simulink model "pv_test"  (R2016a)
settings: Solver=VariableStepAuto  StartTime=0.0  StopTime=0.02  RelTol=1e-3
libraries: powerlib x99, powerlib_meascontrol x30, re_lib x3, simulink x1
settings Model: Creator=Francis Chen  LastModifiedBy=Francis Chen

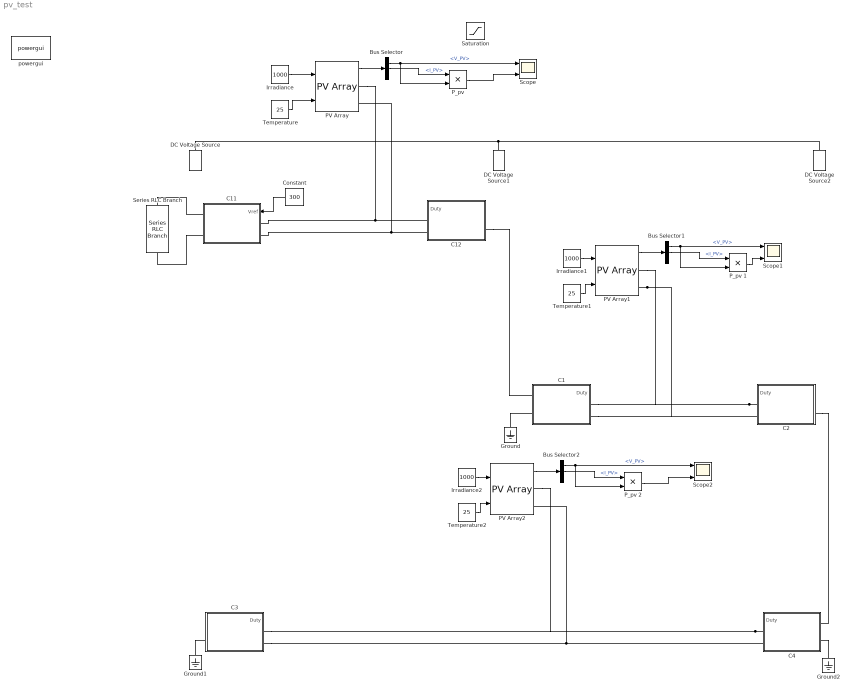
== system pv_test ==
  Bus Selector : BusSelector  OutputSignals=V_PV,I_PV,Irradiance (W/m2)
  Bus Selector1 : BusSelector  OutputSignals=V_PV,I_PV,Irradiance (W/m2)
  Bus Selector2 : BusSelector  OutputSignals=V_PV,I_PV,Irradiance (W/m2)
  C1 : Subsystem
  C11 : Subsystem
  C12 : Subsystem
  C2 : Subsystem
  C3 : Subsystem
  C4 : Subsystem
  Constant : Constant  Value=300
  DC Voltage Source : powerlib/Electrical Sources/DC Voltage Source  Amplitude=100  Measurements=None
  DC Voltage Source1 : powerlib/Electrical Sources/DC Voltage Source  Amplitude=100  Measurements=None
  DC Voltage Source2 : powerlib/Electrical Sources/DC Voltage Source  Amplitude=100  Measurements=None
  Ground : powerlib/Elements/Ground  LConnTagsString=a
  Ground1 : powerlib/Elements/Ground  LConnTagsString=a
  Ground2 : powerlib/Elements/Ground  LConnTagsString=a
  Irradiance : Constant  Value=1000
  Irradiance1 : Constant  Value=1000
  Irradiance2 : Constant  Value=1000
  PV Array : re_lib/Solar/PV Array  Npar=1  Nser=10  PlotType=array @ 1000 W/m2 & specified temperatures  S_vec="[ 1000  500  100 ]"  Temp_C_vec=[25]  ModuleName=1Soltech 1STH-215-P  PlotWhenSelected=off  Pm=213.15  Ncell=60  Voc=36.3  Isc=7.84  Vm=29  Im=7.35  beta_Voc_pc=-0.36099  alpha_Isc_pc=0.102  beta_Voc=-0.13104  alpha_Isc=0.007997  IL=7.8649  I0=2.9259e-10  nI=0.98117  Rsh=313.3991  Rs=0.39383  BAL=off  Tc=1e-6  Tfilter=5e-5
  PV Array1 : re_lib/Solar/PV Array  Npar=1  Nser=10  PlotType=array @ 1000 W/m2 & specified temperatures  S_vec="[ 1000  500  100 ]"  Temp_C_vec="[ 45 25  ]"  ModuleName=1Soltech 1STH-215-P  PlotWhenSelected=off  Pm=213.15  Ncell=60  Voc=36.3  Isc=7.84  Vm=29  Im=7.35  beta_Voc_pc=-0.36099  alpha_Isc_pc=0.102  beta_Voc=-0.13104  alpha_Isc=0.007997  IL=7.8649  I0=2.9259e-10  nI=0.98117  Rsh=313.3991  Rs=0.39383  BAL=off  Tc=1e-6  Tfilter=5e-5
  PV Array2 : re_lib/Solar/PV Array  Npar=1  Nser=10  PlotType=array @ 1000 W/m2 & specified temperatures  S_vec="[ 1000  500  100 ]"  Temp_C_vec="[ 45 25  ]"  ModuleName=1Soltech 1STH-215-P  PlotWhenSelected=off  Pm=213.15  Ncell=60  Voc=36.3  Isc=7.84  Vm=29  Im=7.35  beta_Voc_pc=-0.36099  alpha_Isc_pc=0.102  beta_Voc=-0.13104  alpha_Isc=0.007997  IL=7.8649  I0=2.9259e-10  nI=0.98117  Rsh=313.3991  Rs=0.39383  BAL=off  Tc=1e-6  Tfilter=5e-5
  "P_pv " : Product
  P_pv 1 : Product
  P_pv 2 : Product
  Saturation : Saturate  UpperLimit=1  LowerLimit=0
  Scope : Scope  NumInputPorts=3
  Scope1 : Scope  NumInputPorts=3
  Scope2 : Scope  NumInputPorts=3
  Series RLC Branch : powerlib/Elements/Series RLC Branch  LConnTagsString=__new0  RConnTagsString=__new0  BranchType=R  Resistance=30  Inductance=1e-3  SetiL0=off  InitialCurrent=0  Capacitance=1e-6  Setx0=off  InitialVoltage=0  Measurements=None
  Temperature : Constant  Value=25
  Temperature1 : Constant  Value=25
  Temperature2 : Constant  Value=25
  powergui : powerlib/powergui  Priority=1  SimulationMode=Discrete  SolverType=Tustin  SampleTime=3e-8  frequency=60  SPID=on  DisableSnubberDevices=on  DisableRonSwitches=off  DisableVfSwitches=off  SwTol=0  DisplayEquations=off  Interpol=off  ExternalGateDelay=off  methode=off  Ts=10  FunctionMessages=off  echomessages=off  HookPort=off  EnableUseOfTLC=off  x0status=blocks  frequencyindice=0  Pbase=100e6  ErrMax=1e-4  Iterations=50  UnitsV=kV  UnitsW=MW  buscounter=0  RestoreLinks=warning  ResistiveCurrentMeasurement=off  Frange=[0:2:500]  Ylog=off  Xlog=on  ShowGrid=off  save=off  variable=ZData  structure=0  ZoomFFT=off  StartTime=0.0  cycles=1  DisplayStyle=1  fundamental=60  FreqAxis=off  MaxFrequency=1000  frequencyindicesteady=1  RmsSteady=1  display=off
  wires:
  "P_pv "/1 -> Scope/3
  PV Array/1 -> Bus Selector/1
  Temperature/1 -> PV Array/2
  Irradiance/1 -> PV Array/1
  Bus Selector/1 -> "P_pv "/2, Scope/1  "<V_PV>"
  Bus Selector/2 -> "P_pv "/1  "<I_PV>"
  P_pv 1/1 -> Scope1/3
  PV Array1/1 -> Bus Selector1/1
  Temperature1/1 -> PV Array1/2
  Irradiance1/1 -> PV Array1/1
  Bus Selector1/1 -> P_pv 1/2, Scope1/1  "<V_PV>"
  Bus Selector1/2 -> P_pv 1/1  "<I_PV>"
  P_pv 2/1 -> Scope2/3
  PV Array2/1 -> Bus Selector2/1
  Temperature2/1 -> PV Array2/2
  Irradiance2/1 -> PV Array2/1
  Bus Selector2/1 -> P_pv 2/2, Scope2/1  "<V_PV>"
  Bus Selector2/2 -> P_pv 2/1  "<I_PV>"
  Constant/1 -> C11/1(Vref)
  connections:
  PV Array/RConn1 -- C11/LConn1 -- C12/LConn1
  C12/LConn2 -- C11/LConn2 -- PV Array/RConn2
  C2/LConn1 -- PV Array1/RConn1 -- C1/LConn1
  PV Array1/RConn2 -- C2/LConn2 -- C1/LConn2
  C4/LConn1 -- PV Array2/RConn1 -- C3/LConn1
  C3/LConn2 -- PV Array2/RConn2 -- C4/LConn2
  C12/RConn2 -- C1/RConn1
  C1/RConn2 -- Ground/LConn1
  C3/RConn2 -- Ground1/LConn1
  C2/RConn2 -- C4/RConn1
  C4/RConn2 -- Ground2/LConn1
  DC Voltage Source/LConn1 -- DC Voltage Source2/LConn1 -- DC Voltage Source1/LConn1
  C11/RConn1 -- Series RLC Branch/LConn1
  C11/RConn2 -- Series RLC Branch/RConn1

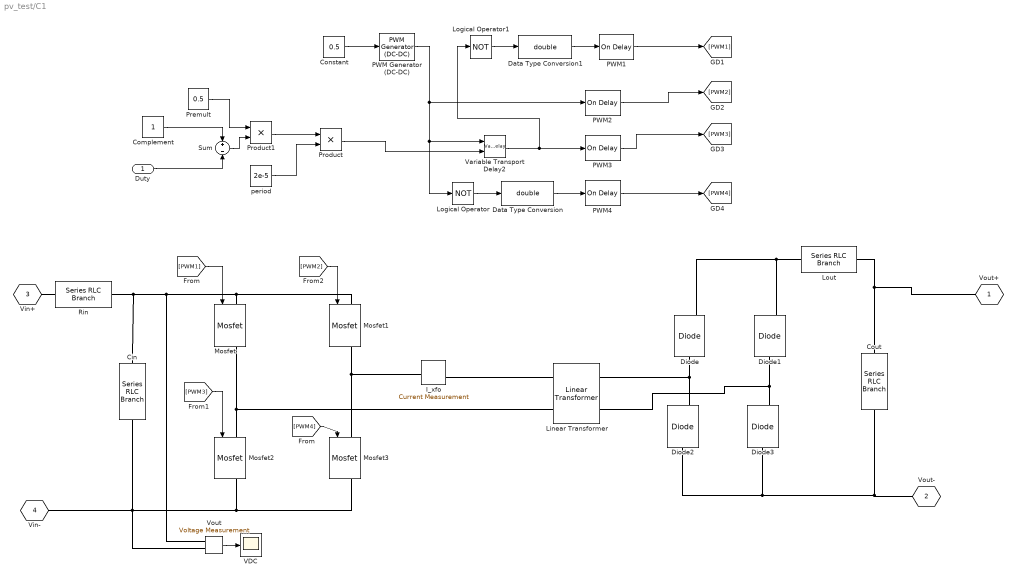
== system pv_test/C1 ==
  Duty : Inport
  Cin : powerlib/Elements/Series RLC Branch  LConnTagsString=__new0  RConnTagsString=__new0  BranchType=C  Resistance=1  Inductance=1e-3  SetiL0=off  InitialCurrent=0  Capacitance=50e-6  Setx0=on  InitialVoltage=300  Measurements=None
  Complement : Constant
  Constant : Constant  Value=0.5
  Cout : powerlib/Elements/Series RLC Branch  LConnTagsString=__new0  RConnTagsString=__new0  BranchType=C  Resistance=0.01  Inductance=1e-3  SetiL0=off  InitialCurrent=0  Capacitance=2e-6  Setx0=on  InitialVoltage=0  Measurements=None
  Data Type Conversion : DataTypeConversion  OutDataTypeStr=double
  Data Type Conversion1 : DataTypeConversion  OutDataTypeStr=double
  Diode{,1..3} (4 alike) : powerlib/Power Electronics/Diode  Ron=0.01  Lon=0  Vf=0.8  IC=0  UseSnubber=off  Rs=1e3  Cs=250e-9  Measurements=on
  I_xfo : powerlib/Measurements/Current Measurement  PhasorSimulation=off  OutputType=Complex  PSBequivalent=0
  Linear Transformer : powerlib/Elements/Linear Transformer  UNITS=SI  NominalPower=[1000,100e3]  winding1=[100 0.2 1e-6]  winding2=[100 0.2 1e-6]  ThreeWindings=off  winding3=[3.15e+05 1.9845e+06 126.34]  RmLm=[50000 1e-3]  Measurements=Winding voltages  DataType=on
  Logical Operator : Logic  Operator=NOT  Inputs=1  AllPortsSameDT=off  OutDataTypeStr=boolean
  Logical Operator1 : Logic  Operator=NOT  Inputs=1  AllPortsSameDT=off  OutDataTypeStr=boolean
  Lout : powerlib/Elements/Series RLC Branch  LConnTagsString=__new0  RConnTagsString=__new0  BranchType=L  Resistance=0.1  Inductance=1e-4  SetiL0=off  InitialCurrent=0  Capacitance=1e-6  Setx0=off  InitialVoltage=0  Measurements=None
  Mosfet : powerlib/Power Electronics/Mosfet  Ron=0.1  Lon=0  Rd=0.01  Vfd=0  IC=0  Rs=inf  Cs=inf  Measurements=on
  Mosfet1 : powerlib/Power Electronics/Mosfet  Ron=0.1  Lon=0  Rd=0.01  Vfd=0  IC=0  Rs=inf  Cs=inf  Measurements=on
  Mosfet2 : powerlib/Power Electronics/Mosfet  Ron=0.1  Lon=0  Rd=0.01  Vfd=0  IC=0  Rs=1e10  Cs=inf  Measurements=on
  Mosfet3 : powerlib/Power Electronics/Mosfet  Ron=0.1  Lon=0  Rd=0.01  Vfd=0  IC=0  Rs=1e10  Cs=inf  Measurements=on
  PWM Generator (DC-DC) : powerlib_meascontrol/Pulse & Signal Generators/PWM Generator (DC-DC)  Fsw=50e3  Ts=0
  PWM{1..4} (4 alike) : powerlib_meascontrol/Logic/On Delay  DelayType=On delay  delay=1e-7  ic=0  Ts=0
  Premult : Constant  Value=0.5
  Product : Product
  Product1 : Product
  Rin : powerlib/Elements/Series RLC Branch  LConnTagsString=__new0  RConnTagsString=__new0  BranchType=R  Resistance=0.1  Inductance=1e-3  SetiL0=off  InitialCurrent=0  Capacitance=1e-6  Setx0=off  InitialVoltage=0  Measurements=None
  Sum : Sum  Inputs=+-
  VDC : Scope
  Variable Transport Delay2 : VariableTransportDelay  MaximumDelay=10  ZeroDelay=on
  Vout : powerlib/Measurements/Voltage Measurement  PhasorSimulation=off  OutputType=Complex  PSBequivalent=0
  "period " : Constant  Value=2e-5
  Vout+ : PMIOPort  Tag=PMCPort  Port=1  Side=Right
  Vout- : PMIOPort  Tag=PMCPort  Port=2  Side=Right
  Vin+ : PMIOPort  Tag=PMCPort  Port=3  Side=Left
  Vin- : PMIOPort  Tag=PMCPort  Port=4  Side=Left
  wires:
  Constant/1 -> PWM Generator (DC-DC)/1
  [PWM1] -> Mosfet/1
  [PWM4] -> Mosfet3/1
  [PWM3] -> Mosfet2/1
  [PWM2] -> Mosfet1/1
  PWM1/1 -> [PWM1]
  PWM3/1 -> [PWM3]
  PWM2/1 -> [PWM2]
  PWM4/1 -> [PWM4]
  PWM Generator (DC-DC)/1 -> PWM2/1, Logical Operator/1, Variable Transport Delay2/1
  Variable Transport Delay2/1 -> Logical Operator1/1, PWM3/1
  Logical Operator/1 -> Data Type Conversion/1
  Data Type Conversion/1 -> PWM4/1
  "period "/1 -> Product/2
  Product/1 -> Variable Transport Delay2/2
  Logical Operator1/1 -> Data Type Conversion1/1
  Data Type Conversion1/1 -> PWM1/1
  Product1/1 -> Product/1
  Premult/1 -> Product1/1
  Complement/1 -> Sum/1
  Sum/1 -> Product1/2
  Duty/1 -> Sum/2
  Vout/1 -> VDC/1
  connections:
  Diode2/RConn1 -- Linear Transformer/RConn1 -- Diode/LConn1
  Diode2/LConn1 -- Cout/RConn1 -- Vout-/RConn1 -- Diode3/LConn1
  Diode3/RConn1 -- Linear Transformer/RConn2 -- Diode1/LConn1
  Vin+/RConn1 -- Rin/LConn1
  Mosfet3/RConn1 -- Mosfet2/RConn1 -- Cin/RConn1 -- Vin-/RConn1 -- Vout/LConn2
  Mosfet/RConn1 -- Linear Transformer/LConn2 -- Mosfet2/LConn1
  Mosfet1/RConn1 -- I_xfo/LConn1 -- Mosfet3/LConn1
  Mosfet1/LConn1 -- Mosfet/LConn1 -- Rin/RConn1 -- Cin/LConn1 -- Vout/LConn1
  Linear Transformer/LConn1 -- I_xfo/RConn1
  Cout/LConn1 -- Lout/RConn1 -- Vout+/RConn1
  Diode1/RConn1 -- Lout/LConn1 -- Diode/RConn1

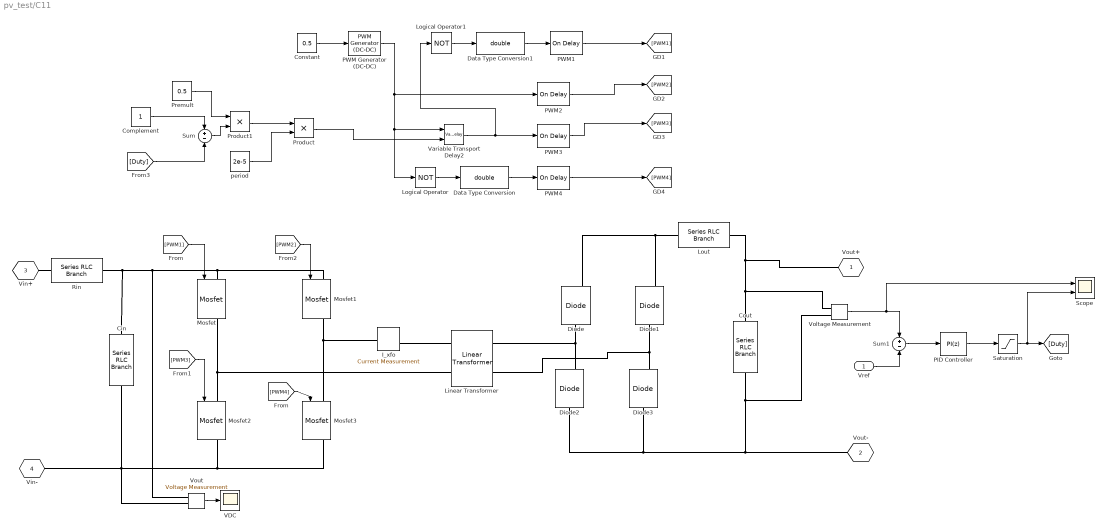
== system pv_test/C11 ==
  Vref : Inport
  Cin : powerlib/Elements/Series RLC Branch  LConnTagsString=__new0  RConnTagsString=__new0  BranchType=C  Resistance=1  Inductance=1e-3  SetiL0=off  InitialCurrent=0  Capacitance=50e-6  Setx0=on  InitialVoltage=300  Measurements=None
  Complement : Constant
  Constant : Constant  Value=0.5
  Cout : powerlib/Elements/Series RLC Branch  LConnTagsString=__new0  RConnTagsString=__new0  BranchType=C  Resistance=0.01  Inductance=1e-3  SetiL0=off  InitialCurrent=0  Capacitance=2e-6  Setx0=on  InitialVoltage=0  Measurements=None
  Data Type Conversion : DataTypeConversion  OutDataTypeStr=double
  Data Type Conversion1 : DataTypeConversion  OutDataTypeStr=double
  Diode{,1..3} (4 alike) : powerlib/Power Electronics/Diode  Ron=0.01  Lon=0  Vf=0.8  IC=0  UseSnubber=off  Rs=1e3  Cs=250e-9  Measurements=on
  I_xfo : powerlib/Measurements/Current Measurement  PhasorSimulation=off  OutputType=Complex  PSBequivalent=0
  Linear Transformer : powerlib/Elements/Linear Transformer  UNITS=SI  NominalPower=[1000,100e3]  winding1=[100 0.2 1e-6]  winding2=[100 0.2 1e-6]  ThreeWindings=off  winding3=[3.15e+05 1.9845e+06 126.34]  RmLm=[50000 1e-3]  Measurements=Winding voltages  DataType=on
  Logical Operator : Logic  Operator=NOT  Inputs=1  AllPortsSameDT=off  OutDataTypeStr=boolean
  Logical Operator1 : Logic  Operator=NOT  Inputs=1  AllPortsSameDT=off  OutDataTypeStr=boolean
  Lout : powerlib/Elements/Series RLC Branch  LConnTagsString=__new0  RConnTagsString=__new0  BranchType=L  Resistance=0.1  Inductance=1e-4  SetiL0=off  InitialCurrent=0  Capacitance=1e-6  Setx0=off  InitialVoltage=0  Measurements=None
  Mosfet : powerlib/Power Electronics/Mosfet  Ron=0.1  Lon=0  Rd=0.01  Vfd=0  IC=0  Rs=inf  Cs=inf  Measurements=on
  Mosfet1 : powerlib/Power Electronics/Mosfet  Ron=0.1  Lon=0  Rd=0.01  Vfd=0  IC=0  Rs=inf  Cs=inf  Measurements=on
  Mosfet2 : powerlib/Power Electronics/Mosfet  Ron=0.1  Lon=0  Rd=0.01  Vfd=0  IC=0  Rs=1e10  Cs=inf  Measurements=on
  Mosfet3 : powerlib/Power Electronics/Mosfet  Ron=0.1  Lon=0  Rd=0.01  Vfd=0  IC=0  Rs=1e10  Cs=inf  Measurements=on
  PID Controller : simulink/Continuous/PID Controller  Controller=PI  TimeDomain=Discrete-time  SampleTime=-1  IntegratorMethod=Forward Euler  FilterMethod=Forward Euler  Form=Parallel  UseFilter=on  ControllerParametersSource=internal  P=-0.01  I=1  D=0  N=100  InitialConditionSource=internal  InitialConditionForIntegrator=0  InitialConditionForFilter=0  ExternalReset=none  LimitOutput=off  UpperSaturationLimit=inf  LowerSaturationLimit=-inf  LinearizeAsGain=on  AntiWindupMode=none  Kb=1  TrackingMode=off  Kt=1  PParamMin=[]  PParamMax=[]  IParamMin=[]  IParamMax=[]  DParamMin=[]  DParamMax=[]  NParamMin=[]  NParamMax=[]  KbParamMin=[]  KbParamMax=[]  KtParamMin=[]  KtParamMax=[]  POutMin=[]  POutMax=[]  IOutMin=[]  IOutMax=[]  DOutMin=[]  DOutMax=[]  NOutMin=[]  NOutMax=[]  KbOutMin=[]  KbOutMax=[]  KtOutMin=[]  KtOutMax=[]  IntegratorOutMin=[]  IntegratorOutMax=[]  FilterOutMin=[]  FilterOutMax=[]  SumOutMin=[]  SumOutMax=[]  SumI1OutMin=[]  SumI1OutMax=[]  SumI2OutMin=[]  SumI2OutMax=[]  SumI3OutMin=[]  SumI3OutMax=[]  SumDOutMin=[]  SumDOutMax=[]  SaturationOutMin=[]  SaturationOutMax=[]  IntegratorContinuousStateAttributes=''  IntegratorStateMustResolveToSignalObject=off  IntegratorRTWStateStorageClass=Auto  FilterContinuousStateAttributes=''  FilterStateMustResolveToSignalObject=off  FilterRTWStateStorageClass=Auto  DifferentiatorICPrevScaledInput=0  DifferentiatorOutMin=[]  DifferentiatorOutMax=[]
  PWM Generator (DC-DC) : powerlib_meascontrol/Pulse & Signal Generators/PWM Generator (DC-DC)  Fsw=50e3  Ts=0
  PWM{1..4} (4 alike) : powerlib_meascontrol/Logic/On Delay  DelayType=On delay  delay=1e-7  ic=0  Ts=0
  Premult : Constant  Value=0.5
  Product : Product
  Product1 : Product
  Rin : powerlib/Elements/Series RLC Branch  LConnTagsString=__new0  RConnTagsString=__new0  BranchType=R  Resistance=0.1  Inductance=1e-3  SetiL0=off  InitialCurrent=0  Capacitance=1e-6  Setx0=off  InitialVoltage=0  Measurements=None
  Saturation : Saturate  UpperLimit=1  LowerLimit=0
  Scope : Scope  NumInputPorts=2
  Sum : Sum  Inputs=+-
  Sum1 : Sum  Inputs=+-
  VDC : Scope
  Variable Transport Delay2 : VariableTransportDelay  MaximumDelay=10  ZeroDelay=on
  Voltage Measurement : powerlib/Measurements/Voltage Measurement  PhasorSimulation=off  OutputType=Complex  PSBequivalent=0
  Vout : powerlib/Measurements/Voltage Measurement  PhasorSimulation=off  OutputType=Complex  PSBequivalent=0
  "period " : Constant  Value=2e-5
  Vout+ : PMIOPort  Tag=PMCPort  Port=1  Side=Right
  Vout- : PMIOPort  Tag=PMCPort  Port=2  Side=Right
  Vin+ : PMIOPort  Tag=PMCPort  Port=3  Side=Left
  Vin- : PMIOPort  Tag=PMCPort  Port=4  Side=Left
  wires:
  Constant/1 -> PWM Generator (DC-DC)/1
  [PWM1] -> Mosfet/1
  [PWM4] -> Mosfet3/1
  [PWM3] -> Mosfet2/1
  [PWM2] -> Mosfet1/1
  PWM1/1 -> [PWM1]
  PWM3/1 -> [PWM3]
  PWM2/1 -> [PWM2]
  PWM4/1 -> [PWM4]
  PWM Generator (DC-DC)/1 -> PWM2/1, Logical Operator/1, Variable Transport Delay2/1
  Variable Transport Delay2/1 -> Logical Operator1/1, PWM3/1
  Logical Operator/1 -> Data Type Conversion/1
  Data Type Conversion/1 -> PWM4/1
  "period "/1 -> Product/2
  Product/1 -> Variable Transport Delay2/2
  Logical Operator1/1 -> Data Type Conversion1/1
  Data Type Conversion1/1 -> PWM1/1
  Product1/1 -> Product/1
  Premult/1 -> Product1/1
  Complement/1 -> Sum/1
  Sum/1 -> Product1/2
  Vout/1 -> VDC/1
  Voltage Measurement/1 -> Scope/1, Sum1/1
  Vref/1 -> Sum1/2
  Sum1/1 -> PID Controller/1
  [Duty] -> Sum/2
  PID Controller/1 -> Saturation/1
  Saturation/1 -> Scope/2, [Duty]
  connections:
  Diode2/RConn1 -- Linear Transformer/RConn1 -- Diode/LConn1
  Diode2/LConn1 -- Voltage Measurement/LConn2 -- Cout/RConn1 -- Vout-/RConn1 -- Diode3/LConn1
  Diode3/RConn1 -- Linear Transformer/RConn2 -- Diode1/LConn1
  Vin+/RConn1 -- Rin/LConn1
  Mosfet3/RConn1 -- Mosfet2/RConn1 -- Cin/RConn1 -- Vin-/RConn1 -- Vout/LConn2
  Mosfet/RConn1 -- Mosfet2/LConn1 -- Linear Transformer/LConn2
  Mosfet1/RConn1 -- Mosfet3/LConn1 -- I_xfo/LConn1
  Mosfet1/LConn1 -- Mosfet/LConn1 -- Rin/RConn1 -- Cin/LConn1 -- Vout/LConn1
  Linear Transformer/LConn1 -- I_xfo/RConn1
  Cout/LConn1 -- Voltage Measurement/LConn1 -- Lout/RConn1 -- Vout+/RConn1
  Diode1/RConn1 -- Lout/LConn1 -- Diode/RConn1

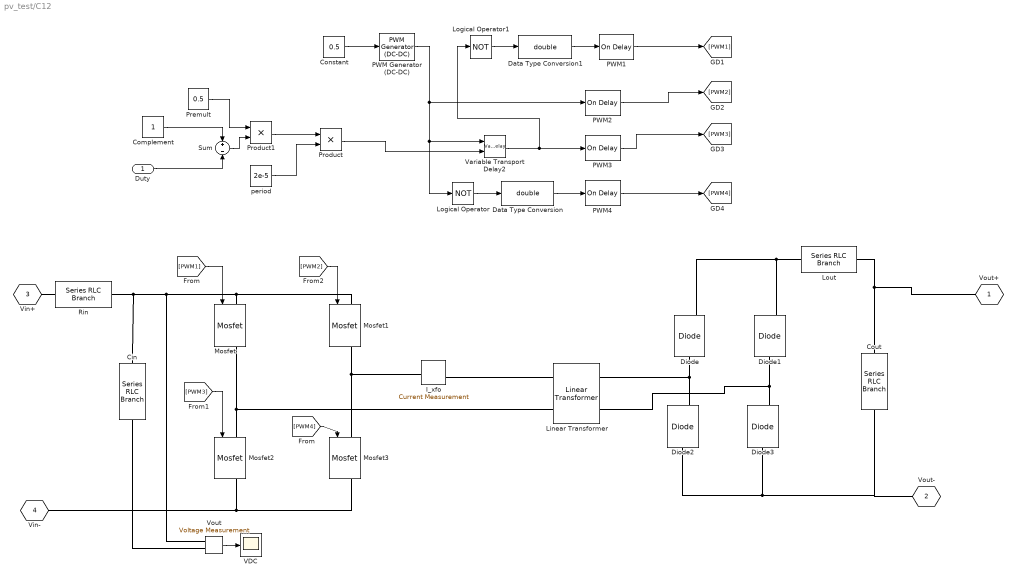
== system pv_test/C12 ==
  Duty : Inport
  Cin : powerlib/Elements/Series RLC Branch  LConnTagsString=__new0  RConnTagsString=__new0  BranchType=C  Resistance=1  Inductance=1e-3  SetiL0=off  InitialCurrent=0  Capacitance=50e-6  Setx0=on  InitialVoltage=300  Measurements=None
  Complement : Constant
  Constant : Constant  Value=0.5
  Cout : powerlib/Elements/Series RLC Branch  LConnTagsString=__new0  RConnTagsString=__new0  BranchType=C  Resistance=0.01  Inductance=1e-3  SetiL0=off  InitialCurrent=0  Capacitance=2e-6  Setx0=on  InitialVoltage=0  Measurements=None
  Data Type Conversion : DataTypeConversion  OutDataTypeStr=double
  Data Type Conversion1 : DataTypeConversion  OutDataTypeStr=double
  Diode{,1..3} (4 alike) : powerlib/Power Electronics/Diode  Ron=0.01  Lon=0  Vf=0.8  IC=0  UseSnubber=off  Rs=1e3  Cs=250e-9  Measurements=on
  I_xfo : powerlib/Measurements/Current Measurement  PhasorSimulation=off  OutputType=Complex  PSBequivalent=0
  Linear Transformer : powerlib/Elements/Linear Transformer  UNITS=SI  NominalPower=[1000,100e3]  winding1=[100 0.2 1e-6]  winding2=[100 0.2 1e-6]  ThreeWindings=off  winding3=[3.15e+05 1.9845e+06 126.34]  RmLm=[50000 1e-3]  Measurements=Winding voltages  DataType=on
  Logical Operator : Logic  Operator=NOT  Inputs=1  AllPortsSameDT=off  OutDataTypeStr=boolean
  Logical Operator1 : Logic  Operator=NOT  Inputs=1  AllPortsSameDT=off  OutDataTypeStr=boolean
  Lout : powerlib/Elements/Series RLC Branch  LConnTagsString=__new0  RConnTagsString=__new0  BranchType=L  Resistance=0.1  Inductance=1e-4  SetiL0=off  InitialCurrent=0  Capacitance=1e-6  Setx0=off  InitialVoltage=0  Measurements=None
  Mosfet : powerlib/Power Electronics/Mosfet  Ron=0.1  Lon=0  Rd=0.01  Vfd=0  IC=0  Rs=inf  Cs=inf  Measurements=on
  Mosfet1 : powerlib/Power Electronics/Mosfet  Ron=0.1  Lon=0  Rd=0.01  Vfd=0  IC=0  Rs=inf  Cs=inf  Measurements=on
  Mosfet2 : powerlib/Power Electronics/Mosfet  Ron=0.1  Lon=0  Rd=0.01  Vfd=0  IC=0  Rs=1e10  Cs=inf  Measurements=on
  Mosfet3 : powerlib/Power Electronics/Mosfet  Ron=0.1  Lon=0  Rd=0.01  Vfd=0  IC=0  Rs=1e10  Cs=inf  Measurements=on
  PWM Generator (DC-DC) : powerlib_meascontrol/Pulse & Signal Generators/PWM Generator (DC-DC)  Fsw=50e3  Ts=0
  PWM{1..4} (4 alike) : powerlib_meascontrol/Logic/On Delay  DelayType=On delay  delay=1e-7  ic=0  Ts=0
  Premult : Constant  Value=0.5
  Product : Product
  Product1 : Product
  Rin : powerlib/Elements/Series RLC Branch  LConnTagsString=__new0  RConnTagsString=__new0  BranchType=R  Resistance=0.1  Inductance=1e-3  SetiL0=off  InitialCurrent=0  Capacitance=1e-6  Setx0=off  InitialVoltage=0  Measurements=None
  Sum : Sum  Inputs=+-
  VDC : Scope
  Variable Transport Delay2 : VariableTransportDelay  MaximumDelay=10  ZeroDelay=on
  Vout : powerlib/Measurements/Voltage Measurement  PhasorSimulation=off  OutputType=Complex  PSBequivalent=0
  "period " : Constant  Value=2e-5
  Vout+ : PMIOPort  Tag=PMCPort  Port=1  Side=Right
  Vout- : PMIOPort  Tag=PMCPort  Port=2  Side=Right
  Vin+ : PMIOPort  Tag=PMCPort  Port=3  Side=Left
  Vin- : PMIOPort  Tag=PMCPort  Port=4  Side=Left
  wires:
  Constant/1 -> PWM Generator (DC-DC)/1
  [PWM1] -> Mosfet/1
  [PWM4] -> Mosfet3/1
  [PWM3] -> Mosfet2/1
  [PWM2] -> Mosfet1/1
  PWM1/1 -> [PWM1]
  PWM3/1 -> [PWM3]
  PWM2/1 -> [PWM2]
  PWM4/1 -> [PWM4]
  PWM Generator (DC-DC)/1 -> PWM2/1, Logical Operator/1, Variable Transport Delay2/1
  Variable Transport Delay2/1 -> Logical Operator1/1, PWM3/1
  Logical Operator/1 -> Data Type Conversion/1
  Data Type Conversion/1 -> PWM4/1
  "period "/1 -> Product/2
  Product/1 -> Variable Transport Delay2/2
  Logical Operator1/1 -> Data Type Conversion1/1
  Data Type Conversion1/1 -> PWM1/1
  Product1/1 -> Product/1
  Premult/1 -> Product1/1
  Complement/1 -> Sum/1
  Sum/1 -> Product1/2
  Duty/1 -> Sum/2
  Vout/1 -> VDC/1
  connections:
  Diode2/RConn1 -- Linear Transformer/RConn1 -- Diode/LConn1
  Diode2/LConn1 -- Cout/RConn1 -- Vout-/RConn1 -- Diode3/LConn1
  Diode3/RConn1 -- Linear Transformer/RConn2 -- Diode1/LConn1
  Vin+/RConn1 -- Rin/LConn1
  Mosfet3/RConn1 -- Vout/LConn2 -- Cin/RConn1 -- Vin-/RConn1 -- Mosfet2/RConn1
  Mosfet/RConn1 -- Linear Transformer/LConn2 -- Mosfet2/LConn1
  Mosfet1/RConn1 -- I_xfo/LConn1 -- Mosfet3/LConn1
  Rin/RConn1 -- Cin/LConn1 -- Vout/LConn1 -- Mosfet1/LConn1 -- Mosfet/LConn1
  Linear Transformer/LConn1 -- I_xfo/RConn1
  Cout/LConn1 -- Vout+/RConn1 -- Lout/RConn1
  Diode1/RConn1 -- Lout/LConn1 -- Diode/RConn1

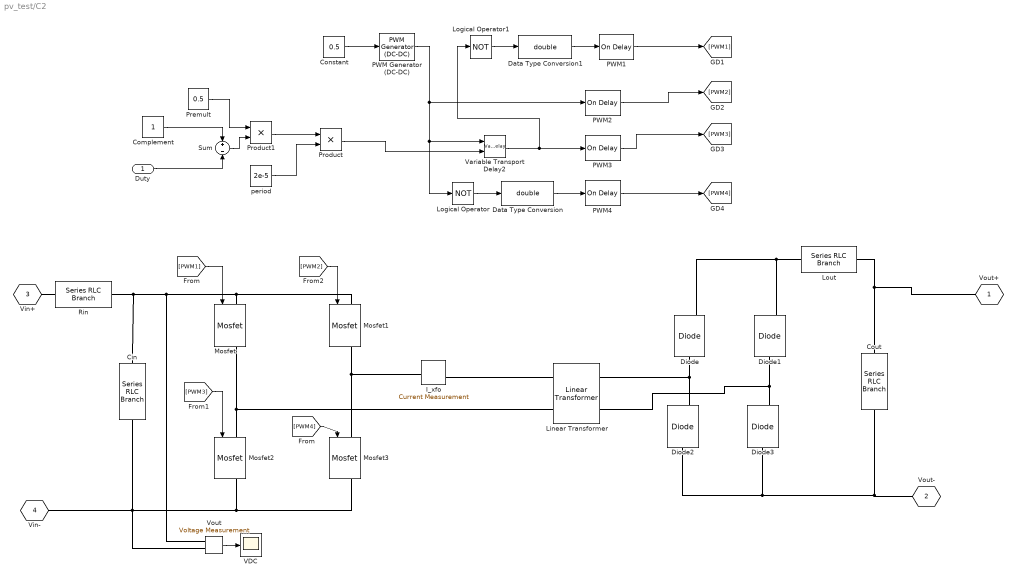
== system pv_test/C2 ==
  Duty : Inport
  Cin : powerlib/Elements/Series RLC Branch  LConnTagsString=__new0  RConnTagsString=__new0  BranchType=C  Resistance=1  Inductance=1e-3  SetiL0=off  InitialCurrent=0  Capacitance=50e-6  Setx0=on  InitialVoltage=300  Measurements=None
  Complement : Constant
  Constant : Constant  Value=0.5
  Cout : powerlib/Elements/Series RLC Branch  LConnTagsString=__new0  RConnTagsString=__new0  BranchType=C  Resistance=0.01  Inductance=1e-3  SetiL0=off  InitialCurrent=0  Capacitance=2e-6  Setx0=on  InitialVoltage=0  Measurements=None
  Data Type Conversion : DataTypeConversion  OutDataTypeStr=double
  Data Type Conversion1 : DataTypeConversion  OutDataTypeStr=double
  Diode{,1..3} (4 alike) : powerlib/Power Electronics/Diode  Ron=0.01  Lon=0  Vf=0.8  IC=0  UseSnubber=off  Rs=1e3  Cs=250e-9  Measurements=on
  I_xfo : powerlib/Measurements/Current Measurement  PhasorSimulation=off  OutputType=Complex  PSBequivalent=0
  Linear Transformer : powerlib/Elements/Linear Transformer  UNITS=SI  NominalPower=[1000,100e3]  winding1=[100 0.2 1e-6]  winding2=[100 0.2 1e-6]  ThreeWindings=off  winding3=[3.15e+05 1.9845e+06 126.34]  RmLm=[50000 1e-3]  Measurements=Winding voltages  DataType=on
  Logical Operator : Logic  Operator=NOT  Inputs=1  AllPortsSameDT=off  OutDataTypeStr=boolean
  Logical Operator1 : Logic  Operator=NOT  Inputs=1  AllPortsSameDT=off  OutDataTypeStr=boolean
  Lout : powerlib/Elements/Series RLC Branch  LConnTagsString=__new0  RConnTagsString=__new0  BranchType=L  Resistance=0.1  Inductance=1e-4  SetiL0=off  InitialCurrent=0  Capacitance=1e-6  Setx0=off  InitialVoltage=0  Measurements=None
  Mosfet : powerlib/Power Electronics/Mosfet  Ron=0.1  Lon=0  Rd=0.01  Vfd=0  IC=0  Rs=inf  Cs=inf  Measurements=on
  Mosfet1 : powerlib/Power Electronics/Mosfet  Ron=0.1  Lon=0  Rd=0.01  Vfd=0  IC=0  Rs=inf  Cs=inf  Measurements=on
  Mosfet2 : powerlib/Power Electronics/Mosfet  Ron=0.1  Lon=0  Rd=0.01  Vfd=0  IC=0  Rs=1e10  Cs=inf  Measurements=on
  Mosfet3 : powerlib/Power Electronics/Mosfet  Ron=0.1  Lon=0  Rd=0.01  Vfd=0  IC=0  Rs=1e10  Cs=inf  Measurements=on
  PWM Generator (DC-DC) : powerlib_meascontrol/Pulse & Signal Generators/PWM Generator (DC-DC)  Fsw=50e3  Ts=0
  PWM{1..4} (4 alike) : powerlib_meascontrol/Logic/On Delay  DelayType=On delay  delay=1e-7  ic=0  Ts=0
  Premult : Constant  Value=0.5
  Product : Product
  Product1 : Product
  Rin : powerlib/Elements/Series RLC Branch  LConnTagsString=__new0  RConnTagsString=__new0  BranchType=R  Resistance=0.1  Inductance=1e-3  SetiL0=off  InitialCurrent=0  Capacitance=1e-6  Setx0=off  InitialVoltage=0  Measurements=None
  Sum : Sum  Inputs=+-
  VDC : Scope
  Variable Transport Delay2 : VariableTransportDelay  MaximumDelay=10  ZeroDelay=on
  Vout : powerlib/Measurements/Voltage Measurement  PhasorSimulation=off  OutputType=Complex  PSBequivalent=0
  "period " : Constant  Value=2e-5
  Vout+ : PMIOPort  Tag=PMCPort  Port=1  Side=Right
  Vout- : PMIOPort  Tag=PMCPort  Port=2  Side=Right
  Vin+ : PMIOPort  Tag=PMCPort  Port=3  Side=Left
  Vin- : PMIOPort  Tag=PMCPort  Port=4  Side=Left
  wires:
  Constant/1 -> PWM Generator (DC-DC)/1
  [PWM1] -> Mosfet/1
  [PWM4] -> Mosfet3/1
  [PWM3] -> Mosfet2/1
  [PWM2] -> Mosfet1/1
  PWM1/1 -> [PWM1]
  PWM3/1 -> [PWM3]
  PWM2/1 -> [PWM2]
  PWM4/1 -> [PWM4]
  PWM Generator (DC-DC)/1 -> PWM2/1, Logical Operator/1, Variable Transport Delay2/1
  Variable Transport Delay2/1 -> Logical Operator1/1, PWM3/1
  Logical Operator/1 -> Data Type Conversion/1
  Data Type Conversion/1 -> PWM4/1
  "period "/1 -> Product/2
  Product/1 -> Variable Transport Delay2/2
  Logical Operator1/1 -> Data Type Conversion1/1
  Data Type Conversion1/1 -> PWM1/1
  Product1/1 -> Product/1
  Premult/1 -> Product1/1
  Complement/1 -> Sum/1
  Sum/1 -> Product1/2
  Duty/1 -> Sum/2
  Vout/1 -> VDC/1
  connections:
  Diode2/RConn1 -- Linear Transformer/RConn1 -- Diode/LConn1
  Diode2/LConn1 -- Cout/RConn1 -- Vout-/RConn1 -- Diode3/LConn1
  Diode3/RConn1 -- Linear Transformer/RConn2 -- Diode1/LConn1
  Vin+/RConn1 -- Rin/LConn1
  Mosfet3/RConn1 -- Mosfet2/RConn1 -- Cin/RConn1 -- Vin-/RConn1 -- Vout/LConn2
  Mosfet/RConn1 -- Linear Transformer/LConn2 -- Mosfet2/LConn1
  Mosfet1/RConn1 -- I_xfo/LConn1 -- Mosfet3/LConn1
  Mosfet1/LConn1 -- Mosfet/LConn1 -- Rin/RConn1 -- Cin/LConn1 -- Vout/LConn1
  Linear Transformer/LConn1 -- I_xfo/RConn1
  Cout/LConn1 -- Lout/RConn1 -- Vout+/RConn1
  Diode1/RConn1 -- Lout/LConn1 -- Diode/RConn1

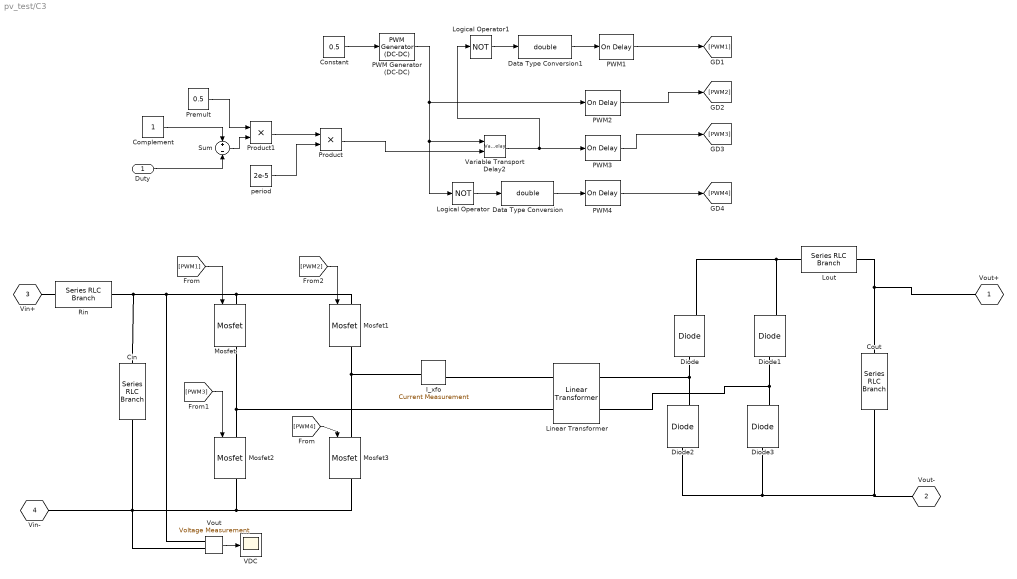
== system pv_test/C3 ==
  Duty : Inport
  Cin : powerlib/Elements/Series RLC Branch  LConnTagsString=__new0  RConnTagsString=__new0  BranchType=C  Resistance=1  Inductance=1e-3  SetiL0=off  InitialCurrent=0  Capacitance=50e-6  Setx0=on  InitialVoltage=300  Measurements=None
  Complement : Constant
  Constant : Constant  Value=0.5
  Cout : powerlib/Elements/Series RLC Branch  LConnTagsString=__new0  RConnTagsString=__new0  BranchType=C  Resistance=0.01  Inductance=1e-3  SetiL0=off  InitialCurrent=0  Capacitance=2e-6  Setx0=on  InitialVoltage=0  Measurements=None
  Data Type Conversion : DataTypeConversion  OutDataTypeStr=double
  Data Type Conversion1 : DataTypeConversion  OutDataTypeStr=double
  Diode{,1..3} (4 alike) : powerlib/Power Electronics/Diode  Ron=0.01  Lon=0  Vf=0.8  IC=0  UseSnubber=off  Rs=1e3  Cs=250e-9  Measurements=on
  I_xfo : powerlib/Measurements/Current Measurement  PhasorSimulation=off  OutputType=Complex  PSBequivalent=0
  Linear Transformer : powerlib/Elements/Linear Transformer  UNITS=SI  NominalPower=[1000,100e3]  winding1=[100 0.2 1e-6]  winding2=[100 0.2 1e-6]  ThreeWindings=off  winding3=[3.15e+05 1.9845e+06 126.34]  RmLm=[50000 1e-3]  Measurements=Winding voltages  DataType=on
  Logical Operator : Logic  Operator=NOT  Inputs=1  AllPortsSameDT=off  OutDataTypeStr=boolean
  Logical Operator1 : Logic  Operator=NOT  Inputs=1  AllPortsSameDT=off  OutDataTypeStr=boolean
  Lout : powerlib/Elements/Series RLC Branch  LConnTagsString=__new0  RConnTagsString=__new0  BranchType=L  Resistance=0.1  Inductance=1e-4  SetiL0=off  InitialCurrent=0  Capacitance=1e-6  Setx0=off  InitialVoltage=0  Measurements=None
  Mosfet : powerlib/Power Electronics/Mosfet  Ron=0.1  Lon=0  Rd=0.01  Vfd=0  IC=0  Rs=inf  Cs=inf  Measurements=on
  Mosfet1 : powerlib/Power Electronics/Mosfet  Ron=0.1  Lon=0  Rd=0.01  Vfd=0  IC=0  Rs=inf  Cs=inf  Measurements=on
  Mosfet2 : powerlib/Power Electronics/Mosfet  Ron=0.1  Lon=0  Rd=0.01  Vfd=0  IC=0  Rs=1e10  Cs=inf  Measurements=on
  Mosfet3 : powerlib/Power Electronics/Mosfet  Ron=0.1  Lon=0  Rd=0.01  Vfd=0  IC=0  Rs=1e10  Cs=inf  Measurements=on
  PWM Generator (DC-DC) : powerlib_meascontrol/Pulse & Signal Generators/PWM Generator (DC-DC)  Fsw=50e3  Ts=0
  PWM{1..4} (4 alike) : powerlib_meascontrol/Logic/On Delay  DelayType=On delay  delay=1e-7  ic=0  Ts=0
  Premult : Constant  Value=0.5
  Product : Product
  Product1 : Product
  Rin : powerlib/Elements/Series RLC Branch  LConnTagsString=__new0  RConnTagsString=__new0  BranchType=R  Resistance=0.1  Inductance=1e-3  SetiL0=off  InitialCurrent=0  Capacitance=1e-6  Setx0=off  InitialVoltage=0  Measurements=None
  Sum : Sum  Inputs=+-
  VDC : Scope
  Variable Transport Delay2 : VariableTransportDelay  MaximumDelay=10  ZeroDelay=on
  Vout : powerlib/Measurements/Voltage Measurement  PhasorSimulation=off  OutputType=Complex  PSBequivalent=0
  "period " : Constant  Value=2e-5
  Vout+ : PMIOPort  Tag=PMCPort  Port=1  Side=Right
  Vout- : PMIOPort  Tag=PMCPort  Port=2  Side=Right
  Vin+ : PMIOPort  Tag=PMCPort  Port=3  Side=Left
  Vin- : PMIOPort  Tag=PMCPort  Port=4  Side=Left
  wires:
  Constant/1 -> PWM Generator (DC-DC)/1
  [PWM1] -> Mosfet/1
  [PWM4] -> Mosfet3/1
  [PWM3] -> Mosfet2/1
  [PWM2] -> Mosfet1/1
  PWM1/1 -> [PWM1]
  PWM3/1 -> [PWM3]
  PWM2/1 -> [PWM2]
  PWM4/1 -> [PWM4]
  PWM Generator (DC-DC)/1 -> PWM2/1, Logical Operator/1, Variable Transport Delay2/1
  Variable Transport Delay2/1 -> Logical Operator1/1, PWM3/1
  Logical Operator/1 -> Data Type Conversion/1
  Data Type Conversion/1 -> PWM4/1
  "period "/1 -> Product/2
  Product/1 -> Variable Transport Delay2/2
  Logical Operator1/1 -> Data Type Conversion1/1
  Data Type Conversion1/1 -> PWM1/1
  Product1/1 -> Product/1
  Premult/1 -> Product1/1
  Complement/1 -> Sum/1
  Sum/1 -> Product1/2
  Duty/1 -> Sum/2
  Vout/1 -> VDC/1
  connections:
  Diode2/RConn1 -- Linear Transformer/RConn1 -- Diode/LConn1
  Diode2/LConn1 -- Cout/RConn1 -- Vout-/RConn1 -- Diode3/LConn1
  Diode3/RConn1 -- Linear Transformer/RConn2 -- Diode1/LConn1
  Vin+/RConn1 -- Rin/LConn1
  Mosfet3/RConn1 -- Mosfet2/RConn1 -- Cin/RConn1 -- Vin-/RConn1 -- Vout/LConn2
  Mosfet/RConn1 -- Linear Transformer/LConn2 -- Mosfet2/LConn1
  Mosfet1/RConn1 -- I_xfo/LConn1 -- Mosfet3/LConn1
  Mosfet1/LConn1 -- Mosfet/LConn1 -- Rin/RConn1 -- Cin/LConn1 -- Vout/LConn1
  Linear Transformer/LConn1 -- I_xfo/RConn1
  Cout/LConn1 -- Lout/RConn1 -- Vout+/RConn1
  Diode1/RConn1 -- Lout/LConn1 -- Diode/RConn1

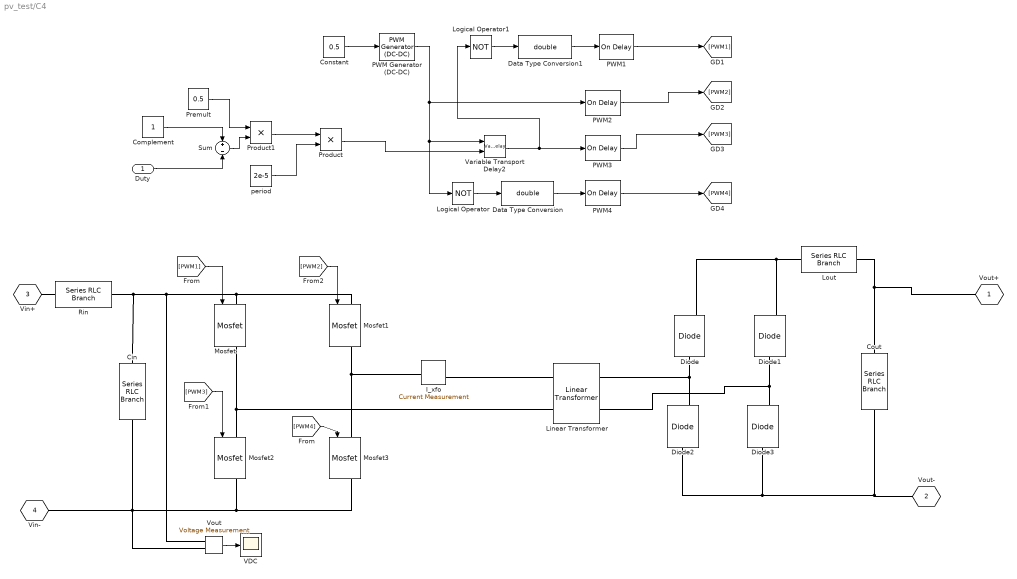
== system pv_test/C4 ==
  Duty : Inport
  Cin : powerlib/Elements/Series RLC Branch  LConnTagsString=__new0  RConnTagsString=__new0  BranchType=C  Resistance=1  Inductance=1e-3  SetiL0=off  InitialCurrent=0  Capacitance=50e-6  Setx0=on  InitialVoltage=300  Measurements=None
  Complement : Constant
  Constant : Constant  Value=0.5
  Cout : powerlib/Elements/Series RLC Branch  LConnTagsString=__new0  RConnTagsString=__new0  BranchType=C  Resistance=0.01  Inductance=1e-3  SetiL0=off  InitialCurrent=0  Capacitance=2e-6  Setx0=on  InitialVoltage=0  Measurements=None
  Data Type Conversion : DataTypeConversion  OutDataTypeStr=double
  Data Type Conversion1 : DataTypeConversion  OutDataTypeStr=double
  Diode{,1..3} (4 alike) : powerlib/Power Electronics/Diode  Ron=0.01  Lon=0  Vf=0.8  IC=0  UseSnubber=off  Rs=1e3  Cs=250e-9  Measurements=on
  I_xfo : powerlib/Measurements/Current Measurement  PhasorSimulation=off  OutputType=Complex  PSBequivalent=0
  Linear Transformer : powerlib/Elements/Linear Transformer  UNITS=SI  NominalPower=[1000,100e3]  winding1=[100 0.2 1e-6]  winding2=[100 0.2 1e-6]  ThreeWindings=off  winding3=[3.15e+05 1.9845e+06 126.34]  RmLm=[50000 1e-3]  Measurements=Winding voltages  DataType=on
  Logical Operator : Logic  Operator=NOT  Inputs=1  AllPortsSameDT=off  OutDataTypeStr=boolean
  Logical Operator1 : Logic  Operator=NOT  Inputs=1  AllPortsSameDT=off  OutDataTypeStr=boolean
  Lout : powerlib/Elements/Series RLC Branch  LConnTagsString=__new0  RConnTagsString=__new0  BranchType=L  Resistance=0.1  Inductance=1e-4  SetiL0=off  InitialCurrent=0  Capacitance=1e-6  Setx0=off  InitialVoltage=0  Measurements=None
  Mosfet : powerlib/Power Electronics/Mosfet  Ron=0.1  Lon=0  Rd=0.01  Vfd=0  IC=0  Rs=inf  Cs=inf  Measurements=on
  Mosfet1 : powerlib/Power Electronics/Mosfet  Ron=0.1  Lon=0  Rd=0.01  Vfd=0  IC=0  Rs=inf  Cs=inf  Measurements=on
  Mosfet2 : powerlib/Power Electronics/Mosfet  Ron=0.1  Lon=0  Rd=0.01  Vfd=0  IC=0  Rs=1e10  Cs=inf  Measurements=on
  Mosfet3 : powerlib/Power Electronics/Mosfet  Ron=0.1  Lon=0  Rd=0.01  Vfd=0  IC=0  Rs=1e10  Cs=inf  Measurements=on
  PWM Generator (DC-DC) : powerlib_meascontrol/Pulse & Signal Generators/PWM Generator (DC-DC)  Fsw=50e3  Ts=0
  PWM{1..4} (4 alike) : powerlib_meascontrol/Logic/On Delay  DelayType=On delay  delay=1e-7  ic=0  Ts=0
  Premult : Constant  Value=0.5
  Product : Product
  Product1 : Product
  Rin : powerlib/Elements/Series RLC Branch  LConnTagsString=__new0  RConnTagsString=__new0  BranchType=R  Resistance=0.1  Inductance=1e-3  SetiL0=off  InitialCurrent=0  Capacitance=1e-6  Setx0=off  InitialVoltage=0  Measurements=None
  Sum : Sum  Inputs=+-
  VDC : Scope
  Variable Transport Delay2 : VariableTransportDelay  MaximumDelay=10  ZeroDelay=on
  Vout : powerlib/Measurements/Voltage Measurement  PhasorSimulation=off  OutputType=Complex  PSBequivalent=0
  "period " : Constant  Value=2e-5
  Vout+ : PMIOPort  Tag=PMCPort  Port=1  Side=Right
  Vout- : PMIOPort  Tag=PMCPort  Port=2  Side=Right
  Vin+ : PMIOPort  Tag=PMCPort  Port=3  Side=Left
  Vin- : PMIOPort  Tag=PMCPort  Port=4  Side=Left
  wires:
  Constant/1 -> PWM Generator (DC-DC)/1
  [PWM1] -> Mosfet/1
  [PWM4] -> Mosfet3/1
  [PWM3] -> Mosfet2/1
  [PWM2] -> Mosfet1/1
  PWM1/1 -> [PWM1]
  PWM3/1 -> [PWM3]
  PWM2/1 -> [PWM2]
  PWM4/1 -> [PWM4]
  PWM Generator (DC-DC)/1 -> PWM2/1, Logical Operator/1, Variable Transport Delay2/1
  Variable Transport Delay2/1 -> Logical Operator1/1, PWM3/1
  Logical Operator/1 -> Data Type Conversion/1
  Data Type Conversion/1 -> PWM4/1
  "period "/1 -> Product/2
  Product/1 -> Variable Transport Delay2/2
  Logical Operator1/1 -> Data Type Conversion1/1
  Data Type Conversion1/1 -> PWM1/1
  Product1/1 -> Product/1
  Premult/1 -> Product1/1
  Complement/1 -> Sum/1
  Sum/1 -> Product1/2
  Duty/1 -> Sum/2
  Vout/1 -> VDC/1
  connections:
  Diode2/RConn1 -- Linear Transformer/RConn1 -- Diode/LConn1
  Diode2/LConn1 -- Cout/RConn1 -- Vout-/RConn1 -- Diode3/LConn1
  Diode3/RConn1 -- Linear Transformer/RConn2 -- Diode1/LConn1
  Vin+/RConn1 -- Rin/LConn1
  Mosfet3/RConn1 -- Mosfet2/RConn1 -- Cin/RConn1 -- Vin-/RConn1 -- Vout/LConn2
  Mosfet/RConn1 -- Linear Transformer/LConn2 -- Mosfet2/LConn1
  Mosfet1/RConn1 -- I_xfo/LConn1 -- Mosfet3/LConn1
  Mosfet1/LConn1 -- Mosfet/LConn1 -- Rin/RConn1 -- Cin/LConn1 -- Vout/LConn1
  Linear Transformer/LConn1 -- I_xfo/RConn1
  Cout/LConn1 -- Lout/RConn1 -- Vout+/RConn1
  Diode1/RConn1 -- Lout/LConn1 -- Diode/RConn1
